simulink model "Hinf_sim"  (R2017a)
settings: Solver=ode23s  StartTime=0.0  StopTime=run_time  FixedStep=0.001  RelTol=1e-3
values from neighbouring files (symbols this model uses):
  Ask = [0 1 0 0 ... (first row only)    [H_inf_ctrl.m]
  Bsk = [0 0 0 0 ... (first row only)    [H_inf_ctrl.m]
  Csk = [0 1 0 0 ... (first row only)    [H_inf_ctrl.m]
  Dsk = zeros(2,4)    [H_inf_ctrl.m]
  exictation = 1    [H_inf_ctrl.m]    (also in Hinf_control.m = 0; chassis_passive.m = 0; chassis_skyhook.m = 0)
  f = 1    [H_inf_ctrl.m]    (also in Hinf_control.m = 1.1792; chassis_passive.m = 8; chassis_skyhook.m = 1.17615502945)
undefined symbols (not defined in the file or in its folder): Ainf, Binf, Cinf, Dinf
settings Model: Creator=signat  LastModifiedBy=simonignat
settings DataIOCC: LimitDataPoints=on  SaveFormat=Array
settings OptimizationCC: BlockReduction=off  BooleanDataType=off  LifeSpan=inf
settings DebuggingCC: SaveWithParameterizedLinksMsg=none  UnderspecifiedInitializationDetection=Classic  MergeDetectMultiDrivingBlocksExec=none  SignalResolutionControl=TryResolveAllWithWarning  SFUnexpectedBacktrackingDiag=warning  SFNoUnconditionalDefaultTransitionDiag=warning  SFExecutionAtInitializationDiag=none
settings HardwareCC: ProdBitPerPointer=32  ProdBitPerSizeT=32  ProdBitPerPtrDiffT=32  ProdLargestAtomicFloat=None  ProdIntDivRoundTo=Undefined  ProdEndianess=Unspecified  ProdWordSize=32  ProdHWDeviceType=32-bit Generic  TargetUnknown=on
settings ModelReferenceCC: PropagateSignalLabelsOutOfModel=off
settings GRTTargetCC: TargetLangStandard=C89/C90 (ANSI)  GeneratePreprocessorConditionals=Disable all
settings ConfigComp: CovMetricSettings=dw  CovHtmlReporting=on  CovSaveCumulativeToWorkspaceVar=on  CovSaveSingleToWorkspaceVar=on  CovExternalEMLEnable=off  CovSFcnEnable=off

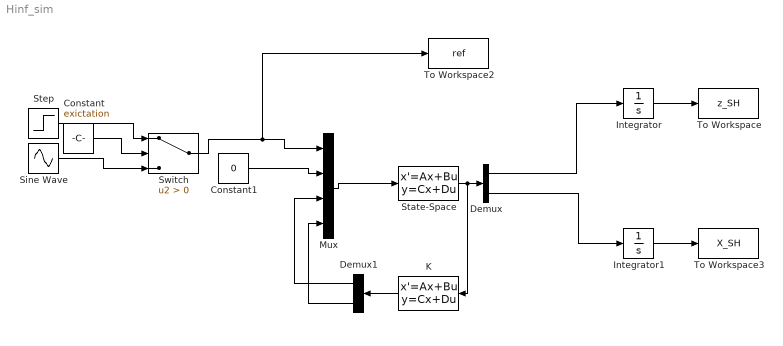
== system Hinf_sim ==
  Constant : Constant  Value=exictation
  Constant1 : Constant  Value=0
  Demux : Demux  Outputs=2
  Demux1 : Demux  Outputs=2
  Integrator : Integrator
  Integrator1 : Integrator
  K : StateSpace  A=Ainf  B=Binf  C=Cinf  D=Dinf  X0=0
  Mux : Mux
  Sine Wave : Sin  Amplitude=0.01  Frequency=f*2*pi  SampleTime=0
  State-Space : StateSpace  A=Ask  B=Bsk  C=Csk  D=Dsk  X0=0
  Step : Step  After=0.03  SampleTime=0
  Switch : Switch  Criteria=u2 > Threshold
  To Workspace : ToWorkspace  VariableName=z_SH  SaveFormat=Timeseries  SampleTime=-1
  To Workspace2 : ToWorkspace  VariableName=ref  SaveFormat=Timeseries  SampleTime=-1
  To Workspace3 : ToWorkspace  VariableName=X_SH  SaveFormat=Timeseries  SampleTime=-1
  wires:
  Step/1 -> Switch/1
  Sine Wave/1 -> Switch/3
  Constant/1 -> Switch/2
  Mux/1 -> State-Space/1
  Switch/1 -> To Workspace2/1, Mux/1
  Constant1/1 -> Mux/2
  State-Space/1 -> K/1, Demux/1
  Demux/1 -> Integrator/1
  Demux/2 -> Integrator1/1
  Integrator/1 -> To Workspace/1
  Integrator1/1 -> To Workspace3/1
  K/1 -> Demux1/1
  Demux1/2 -> Mux/4
  Demux1/1 -> Mux/3
